simulink model "IfElseIf_StateFlow"  (R2020a)
settings: Solver=FixedStepDiscrete  StartTime=0.0  StopTime=10.0  FixedStep=1  RelTol=1e-3
libraries: simulink x1
settings Model: Creator=ashok  LastModifiedBy=ashok

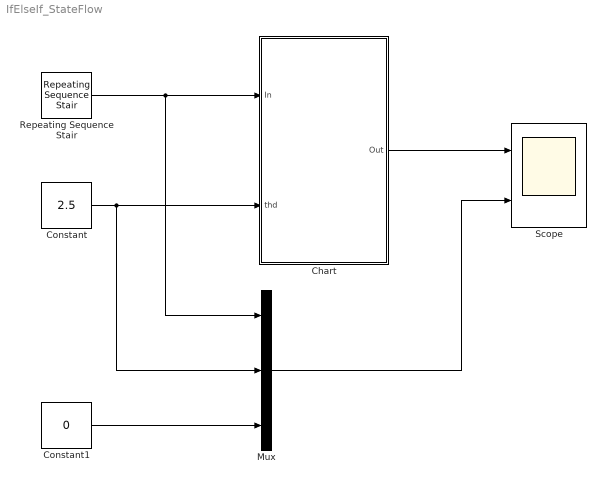
== system IfElseIf_StateFlow ==
  Chart : Stateflow chart  TreatAsAtomicUnit=on
  Constant : Constant  Value=2.5
  Constant1 : Constant  Value=0
  Mux : Mux  Inputs=3
  Repeating Sequence Stair : simulink/Sources/Repeating Sequence Stair  OutValues=[3 1 4 -2 1].'  tsamp=-1  OutMin=[]  OutMax=[]  OutDataTypeStr=double  OutputDataTypeScalingMode=double  OutDataType=fixdt(0,8)  ConRadixGroup=Best Precision: Vector-wise  OutScaling=2^-12
  Scope : Scope  NumInputPorts=2
  wires:
  Constant/1 -> Mux/2, Chart/2(thd)
  Repeating Sequence Stair/1 -> Mux/1, Chart/1(In)
  Constant1/1 -> Mux/3
  Chart/1(Out) -> Scope/1
  Mux/1 -> Scope/2

== stateflow chart IfElseIf_StateFlow/Chart ==
  (default) -> (junction 4)
  (junction 4) -> (junction 8) [order 1] : [In>thd]
  (junction 4) -> (junction 6) [order 2]
  (junction 8) -> (junction 10) : {Out = 1;}
  (junction 6) -> (junction 12) [order 1] : [In>0]
  (junction 6) -> (junction 16) [order 2] : {Out=-1;}
  (junction 12) -> (junction 14) : {Out=0;}
  (junction 14) -> (junction 16)
  (junction 10) -> (junction 14)
  data: In input; thd input; Out output
